simulink model "untitled4"  (Simulink 4.00)
settings: Solver=ode45  StartTime=0.0  StopTime=30  RelTol=1e-3
libraries: cstblocks x4
settings Model: LastModifiedBy=Хозяин  RTWOptions="-aEnforceIntegerDowncast=1 -aExtMode=0 -aFoldNonRolledExpr=1 -aForceParamTrailComments=0 -aGenerateComments=1 -aIgnoreCustomStorageClasses=1 -aIncHierarchyInIds=0 -aInlineInvariantSignals=0 -aLocalBlockOutputs=1 -aLogVarNameModifier=\"rt_\" -aRTWVerbose=1 -aRollThreshold=5 -aShowEliminatedStatements=1"

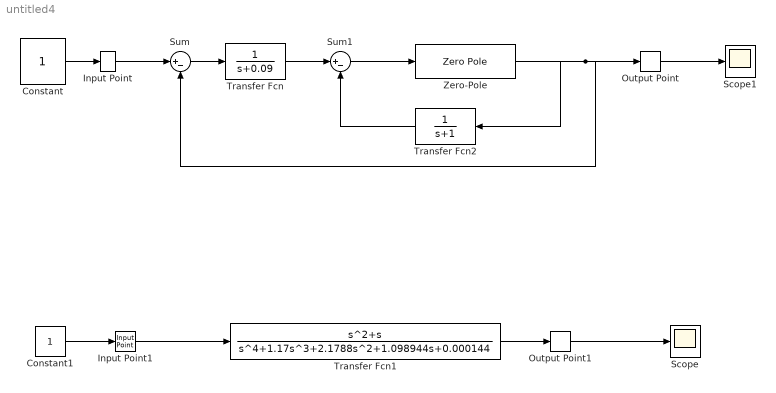
== system untitled4 ==
  Constant : Constant  Value=1
  Constant1 : Constant  Value=1
  Input Point : cstblocks/Input Point
  Input Point1 : cstblocks/Input Point
  Output Point : cstblocks/Output Point
  Output Point1 : cstblocks/Output Point
  Scope : Scope
      settings: TimeRange=auto  YMin=-5  YMax=5  SaveToWorkspace=off  SaveName=ScopeData  LimitDataPoints=on  MaxDataPoints=5000
  Scope1 : Scope
      settings: TimeRange=auto  YMin=-5  YMax=5  SaveToWorkspace=off  LimitDataPoints=on  MaxDataPoints=5000
  Sum : Sum  Inputs=|+-  SaturateOnIntegerOverflow=on
  Sum1 : Sum  Inputs=|+-  SaturateOnIntegerOverflow=on
  Transfer Fcn : TransferFcn  Numerator=[1]  Denominator=[1 0.09]  AbsoluteTolerance=auto  Realization=auto
  Transfer Fcn1 : TransferFcn  Numerator=[1 1 0]  Denominator=[1 1.17 2.1788 1.098944 0.000144]  AbsoluteTolerance=auto  Realization=auto
  Transfer Fcn2 : TransferFcn  Orientation=left  Numerator=[1]  Denominator=[1 1]  AbsoluteTolerance=auto  Realization=auto
  Zero-Pole : ZeroPole  Zeros=[0]  Poles=[-0.04 -0.04]  Gain=[1]  AbsoluteTolerance=auto
  wires:
  Sum/1 -> Transfer Fcn/1
  Transfer Fcn/1 -> Sum1/1
  Sum1/1 -> Zero-Pole/1
  Zero-Pole/1 -> Transfer Fcn2/1, Sum/2, Output Point/1
  Transfer Fcn2/1 -> Sum1/2
  Constant/1 -> Input Point/1
  Input Point/1 -> Sum/1
  Output Point/1 -> Scope1/1
  Constant1/1 -> Input Point1/1
  Input Point1/1 -> Transfer Fcn1/1
  Transfer Fcn1/1 -> Output Point1/1
  Output Point1/1 -> Scope/1
